simulink library "WECSim_Lib"  (R2014b)
settings: Solver=ode45  StartTime=0.0  StopTime=10.0  RelTol=1e-3
undefined symbols (not defined in the file): body, constraint, pto, simu, waves, X, Y, Z
libraries: nesl_utility x178, sm_lib x59, vrlib x12
(part 1 of 6)
settings Model: Creator=cmichel  LastModifiedBy=yyu

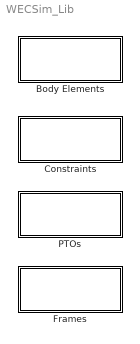
== system WECSim_Lib ==
  Body Elements : Subsystem
      mask Display: text(0,0,' ')
  Constraints : Subsystem
      mask Display: text(0,0,' ')
  Frames : Subsystem
      mask Display: text(0,0,' ')
  PTOs : Subsystem
      mask Display: text(0,0,' ')

== system WECSim_Lib/Body Elements ==
  Rigid Body : Subsystem  mask(BodyElements){body=body(1)}
      mask prompts: body "Body Name:"
      mask help: This block represents a rigid body. The variable name input below must be 'body(i)' where i=1,2,...
      mask init:
      | if exist('body','var')
      |     % geometry file name
      |     h=[gcb '/Structure/Body Properties'];
      |     geomFile=body.geometryFile;
      |     set_param(h,'ExtGeomFileName',geomFile);
      |     % toWorkSpace: outputs
      |     h=[gcb '/To Workspace'];
      |     responseName=['body' num2str(body.bodyNumber) '_out'];
      |     set_param(h,'VariableName',responseName);
      |     % toWorkSpace: hydrostatic pressures
      |     h=[gcb '/Hydrostatic Restoring Force Calculation/Linear and Nonlinear Restoring Force Variant Subsystem/Nonlinear Hydrostatic Restoring Force/To Workspace1'];
      |     responseName=['body' num2str(body.bodyNumber) '_hspressure_out'];
      |     set_param(h,'VariableName',responseName); 
      |     % toWorkSpace: wave pressures (non-linear Freude-Krylov)
      |     h=[gcb '/Wave Diffraction and Excitation Force Calculation/Nonlinear FK Force Variant Subsystem/With Nonlinear FroudeKrylov Force/To Workspace'];
      |     responseName=['body' num2str(body.bodyNumber) '_wavenonlinearpressure_out'];
      |     set_param(h,'VariableName',responseName);
      |     % toWorkSpace: wave pressures (linear Freude-Krylov)
      |     h=[gcb '/Wave Diffraction and Excitation Force Calculation/Nonlinear FK Force Variant Subsystem/With Nonlinear FroudeKrylov Force/To Workspace1'];
      |     responseName=['body' num2str(body.bodyNumber) '_wavelinearpressure_out'];
      |     set_param(h,'VariableName',responseName);
      |     % position GoTo 
      |     h=[gcb '/Goto'];
      |     responseName=['disp' num2str(body.bodyNumber)];
      |     set_param(h,'GotoTag',responseName);
      |     % position From
      |     h=[gcb '/From'];
      |     responseName=['disp' num2str(body.bodyNumber)];
      |     set_param(h,'GotoTag',responseName);
      |     % velocity GoTo 
      |     h=[gcb '/Goto1'];
      |     responseName=['vel' num2str(body.bodyNumber)];
      |     set_param(h,'GotoTag',responseName);
      |     % velocity From 
      |     h=[gcb '/From1'];
      |     responseName=['vel' num2str(body.bodyNumber)];
      |     set_param(h,'GotoTag',responseName);
      |     % acceleration GoTo 
      |     h=[gcb '/Goto2'];
      |     responseName=['acc' num2str(body.bodyNumber)];
      |     set_param(h,'GotoTag',responseName);
      |     % acceleration From 
      |     h=[gcb '/From2'];
      |     responseName=['acc' num2str(body.bodyNumber)];
      |     set_param(h,'GotoTag',responseName);
      | end
      | clear bc h geomFile responseName
      settings: AttributesFormatString=%<body>

== system WECSim_Lib/Constraints ==
  Fixed : Subsystem  mask(Constraints){constraint=constraint(1)}
      mask prompts: constraint "Constraint Name:"
      mask help:
      | Does not allow any motion. The variable name input below must be 'constraint(i)' where i=1,2,...
      |
      | constraint(i) must be defined in the input file with the following fields:
      |     .name              = a string
      |     .loc (optional)    = a 3x1 vector [x y z] in m. Default = [0 0 0]
      | The name string is used as the variable name for the output power and as such must comply with all of Matlab's variable naming rules.
      mask init:
      | if exist('constraint','var')
      |     h=[gcb '/output'];
      |     responseName=['constraint' num2str(constraint.constraintNum) '_out'];
      |     set_param(h,'VariableName',responseName);
      | end
      | 
      | constraint.checkLoc('W');
      settings: AttributesFormatString=%<constraint>
  Floating (3DOF) : Subsystem  mask(Constraints){constraint=constraint(1)}
      mask prompts: constraint "Constraint Name:"
      mask help:
      | Allows body to be free floating (motion in Surge, Heave, and Pitch). The variable name input below must be 'constraint(i)' where i=1,2,...
      |
      | constraint(i) must be defined in the input file with the following fields:
      |     .name              = a string
      |     .loc (optional)    = a 3x1 vector [x y z] in m. Default = [0 0 0]
      |
      | The name string is used as the variable name for the output power and as such must comply with all of Matlab's variable naming rules.
      mask init:
      | if exist('constraint','var')
      |     h=[gcb '/output'];
      |     responseName=['constraint' num2str(constraint.constraintNum) '_out'];
      |     set_param(h,'VariableName',responseName);
      | end
      | 
      | constraint.checkLoc('W');
      settings: AttributesFormatString=%<constraint>
  Floating (6DOF) : Subsystem  mask(Constraints){constraint=constraint(1)}
      mask prompts: constraint "Constraint Name:"
      mask help:
      | Allows body to be free floating (all 6 DOFs). The variable name input below must be 'constraint(i)' where i=1,2,...
      |
      | constraint(i) must be defined in the input file with the following fields:
      |     .name              = a string
      |     .loc (optional)    = a 3x1 vector [x y z] in m. Default = [0 0 0]
      |
      | The name string is used as the variable name for the output power and as such must comply with all of Matlab's variable naming rules.
      mask init: same as WECSim_Lib/Constraints/Floating (3DOF)
      settings: AttributesFormatString=%<constraint>
  Heave : Subsystem  mask(Constraints){constraint=constraint(1)}
      mask prompts: constraint "Constraint Name:"
      mask help:
      | Constrains motion to Heave translation only.The variable name input below must be 'constraint(i)' where i=1,2,...
      |
      | constraint(i) must be defined in the input file with the following fields:
      |     .name              = a string
      |     .loc (optional)    = a 3x1 vector [x y z] in m. Default = [0 0 0]
      | The name string is used as the variable name for the output power and as such must comply with all of Matlab's variable naming rules.
      mask init: same as WECSim_Lib/Constraints/Fixed
      settings: AttributesFormatString=%<constraint>
  Pitch : Subsystem  mask(Constraints){constraint=constraint(1)}
      mask prompts: constraint "Constraint Name:"
      mask help:
      | Constrains motion to Pitch rotation only. The variable name input below must be 'constraint(i)' where i=1,2,...
      |
      | constraint(i) must be defined in the input file with the following fields:
      |     .name   = a string
      |     .loc    = a 3x1 vector [x y z] in m
      |
      | The name string is used as the variable name for the output power and as such must comply with all of Matlab's variable naming rules.
      mask init:
      | if exist('constraint','var')
      |     h=[gcb '/output'];
      |     responseName=['constraint' num2str(constraint.constraintNum) '_out'];
      |     set_param(h,'VariableName',responseName);
      | end
      | 
      | constraint.checkLoc('E');
      settings: AttributesFormatString=%<constraint>
  Surge : Subsystem  mask(Constraints){constraint=constraint(1)}
      mask prompts: constraint "Constraint Name:"
      mask help:
      | Constrains motion to Surge translation only.The variable name input below must be 'constraint(i)' where i=1,2,...
      |
      | constraint(i) must be defined in the input file with the following fields:
      |     .name              = a string
      |     .loc (optional)    = a 3x1 vector [x y z] in m. Default = [0 0 0]
      |
      | The name string is used as the variable name for the output power and as such must comply with all of Matlab's variable naming rules.
      mask init: same as WECSim_Lib/Constraints/Fixed
      settings: AttributesFormatString=%<constraint>

== system WECSim_Lib/Frames ==
  Global Reference Frame : Subsystem  mask(Frames){waves=waves, simu=simu}
      mask prompts: waves "Wave Class Name"; simu "Simulation Class Name"
      mask help:
      | This block contains Global References, including solver configurations, free surface and seabed description, and simulation time.
      | It uses the following fields from the Simulation and Wave classes:
      |
      | Simulation Class:
      |     .endTime
      |     .dt
      |     .domainSize
      |
      | Wave Class:
      |     .waterDepth

== system WECSim_Lib/PTOs ==
  Rotational PTO (Local RY) : Subsystem  mask(PTO){pto=pto(1)}
      mask prompts: pto "PTO Name:"
      mask help:
      | This PTO constrains the follower (F) to only rotate about the Y-axis of the base (B), and applies a PTO stiffness and damping value. The variable name input below must be 'pto(i)' where i=1,2,...
      |
      | pto(i) must be defined in the input file with the following fields:
      |     .name   = a string
      |     .k      = a scalar in N*m/radians
      |     .c      = a scalar in N*m/(radians/s)
      |     .loc    = a 3x1 vector [x y z] in m
      |
      | The name string is used as the variable name for the output power and as such must comply with all of Matlab's variable naming rules.
      mask init:
      | if exist('pto','var')
      |     h=[gcb '/output'];
      |     responseName=['pto' num2str(pto.ptoNum) '_out'];
      |     set_param(h,'VariableName',responseName);
      | end
      | 
      | pto.checkLoc('E');
      settings: AttributesFormatString=%<pto>
  Rotational PTO Prescribed Motion (Local RY) : Subsystem  mask(PTO){pto=pto(1)}
      mask prompts: pto "PTO Name:"
      mask help:
      | This PTO constrains the follower (F) to only rotate about the Y-axis of the base (B), and applies a PTO stiffness and damping value. The variable name input below must be 'pto(i)' where i=1,2,...
      |
      | pto(i) must be defined in the input file with the following fields:
      |     .name   = a string
      |     .k      = a scalar in N*m/radians
      |     .c      = a scalar in N*m/(radians/s)
      |     .loc    = a 3x1 vector [x y z] in m
      |
      | The name string is used as the variable name for the output power and as such must comply with all of Matlab's variable naming rules.
      mask init:
      | if exist('pto','var')
      |     h=[gcb '/output'];
      |     responseName=['pto' num2str(pto.ptoNum) '_out'];
      |     set_param(h,'VariableName',responseName);
      | end
      | 
      | pto.checkLoc('E');
      settings: AttributesFormatString=%<pto>
  Rotational PTO UD Torque (Local RY) : Subsystem  mask(PTO){pto=pto(1)}
      mask prompts: pto "PTO Name:"
      mask help:
      | This PTO constrains the follower (F) to only rotate about the Y-axis of the base (B), and applies a PTO stiffness and damping value. The variable name input below must be 'pto(i)' where i=1,2,...
      |
      | pto(i) must be defined in the input file with the following fields:
      |     .name   = a string
      |     .k      = a scalar in N*m/radians
      |     .c      = a scalar in N*m/(radians/s)
      |     .loc    = a 3x1 vector [x y z] in m
      |
      | The name string is used as the variable name for the output power and as such must comply with all of Matlab's variable naming rules.
      mask init:
      | if exist('pto','var')
      |     h=[gcb '/output'];
      |     responseName=['pto' num2str(pto.ptoNum) '_out'];
      |     set_param(h,'VariableName',responseName);
      | end
      | 
      | pto.checkLoc('E');
      settings: AttributesFormatString=%<pto>
  Translational PTO (Local X) : Subsystem  mask(PTO){pto=pto(1)}
      mask prompts: pto "PTO Name:"
      mask help:
      | This PTO constrains the follower (F) to only move along the X-direction of the base (B), and applies a PTO stiffness and damping value. The variable name input below must be 'pto(i)' where i=1,2,...
      |
      | pto(i) must be defined in the input file with the following fields:
      |     .name              = a string
      |     .k                 = a scalar in N/m
      |     .c                 = a scalar in N/(m/s)
      |     .loc (optional)    = a 3x1 vector [x y z] in m. Default = [0 0 0]
      | The name string is used as the variable name for the output power and as such must comply with all of Matlab's variable naming rules.
      mask init:
      | if exist('pto','var')
      |     h=[gcb '/output'];
      |     responseName=['pto' num2str(pto.ptoNum) '_out'];
      |     set_param(h,'VariableName',responseName);
      | end
      | 
      | pto.checkLoc('W');
      settings: AttributesFormatString=%<pto>
  Translational PTO (Local Z) : Subsystem  mask(PTO){pto=pto(1)}
      mask prompts: pto "PTO Name:"
      mask help:
      | This PTO constrains the follower (F) to only move along the Z-direction of the base (B), and applies a PTO stiffness and damping value. The variable name input below must be 'pto(i)' where i=1,2,...
      |
      | pto(i) must be defined in the input file with the following fields:
      |     .name               = a string
      |     .k                  = a scalar in N/m
      |     .c                  = a scalar in N/(m/s)
      |     .loc (optional)     = a 3x1 vector [x y z] in m. Default = [0 0 0]
      |
      | The name string is used as the variable name for the output power and as such must comply with all of Matlab's variable naming rules.
      mask init:
      | if exist('pto','var')
      |     h=[gcb '/output'];
      |     responseName=['pto' num2str(pto.ptoNum) '_out'];
      |     set_param(h,'VariableName',responseName);
      | end
      | 
      | pto.checkLoc('W');
      settings: AttributesFormatString=%<pto>
  Translational PTO Prescribed Motion (Local X) : Subsystem  mask(PTO){pto=pto(1)}
      mask prompts: pto "PTO Name:"
      mask help:
      | This PTO constrains the follower (F) to only move along the X-direction of the base (B), and applies a PTO stiffness and damping value. The variable name input below must be 'pto(i)' where i=1,2,...
      |
      | pto(i) must be defined in the input file with the following fields:
      |     .name              = a string
      |     .k                 = a scalar in N/m
      |     .c                 = a scalar in N/(m/s)
      |     .loc (optional)    = a 3x1 vector [x y z] in m. Default = [0 0 0]
      | The name string is used as the variable name for the output power and as such must comply with all of Matlab's variable naming rules.
      mask init:
      | if exist('pto','var')
      |     h=[gcb '/output'];
      |     responseName=['pto' num2str(pto.ptoNum) '_out'];
      |     set_param(h,'VariableName',responseName);
      | end
      | 
      | pto.checkLoc('W');
      settings: AttributesFormatString=%<pto>
  Translational PTO Prescribed Motion (Local Z) : Subsystem  mask(PTO){pto=pto(1)}
      mask prompts: pto "PTO Name:"
      mask help:
      | This PTO constrains the follower (F) to only move along the Z-direction of the base (B), and applies a PTO stiffness and damping value. The variable name input below must be 'pto(i)' where i=1,2,...
      |
      | pto(i) must be defined in the input file with the following fields:
      |     .name               = a string
      |     .k                  = a scalar in N/m
      |     .c                  = a scalar in N/(m/s)
      |     .loc (optional)     = a 3x1 vector [x y z] in m. Default = [0 0 0]
      |
      | The name string is used as the variable name for the output power and as such must comply with all of Matlab's variable naming rules.
      mask init:
      | if exist('pto','var')
      |     h=[gcb '/output'];
      |     responseName=['pto' num2str(pto.ptoNum) '_out'];
      |     set_param(h,'VariableName',responseName);
      | end
      | 
      | pto.checkLoc('W');
      settings: AttributesFormatString=%<pto>
  Translational PTO UD Force (Local X) : Subsystem  mask(PTO){pto=pto(1)}
      mask prompts: pto "PTO Name:"
      mask help:
      | This PTO constrains the follower (F) to only move along the X-direction of the base (B), and applies a PTO stiffness and damping value. The variable name input below must be 'pto(i)' where i=1,2,...
      |
      | pto(i) must be defined in the input file with the following fields:
      |     .name              = a string
      |     .k                 = a scalar in N/m
      |     .c                 = a scalar in N/(m/s)
      |     .loc (optional)    = a 3x1 vector [x y z] in m. Default = [0 0 0]
      | The name string is used as the variable name for the output power and as such must comply with all of Matlab's variable naming rules.
      mask init:
      | if exist('pto','var')
      |     h=[gcb '/output'];
      |     responseName=['pto' num2str(pto.ptoNum) '_out'];
      |     set_param(h,'VariableName',responseName);
      | end
      | 
      | pto.checkLoc('W');
      settings: AttributesFormatString=%<pto>
  Translational PTO UD Force (Local Z) : Subsystem  mask(PTO){pto=pto(1)}
      mask prompts: pto "PTO Name:"
      mask help:
      | This PTO constrains the follower (F) to only move along the Z-direction of the base (B), and applies a PTO stiffness and damping value. The variable name input below must be 'pto(i)' where i=1,2,...
      |
      | pto(i) must be defined in the input file with the following fields:
      |     .name               = a string
      |     .k                  = a scalar in N/m
      |     .c                  = a scalar in N/(m/s)
      |     .loc (optional)     = a 3x1 vector [x y z] in m. Default = [0 0 0]
      |
      | The name string is used as the variable name for the output power and as such must comply with all of Matlab's variable naming rules.
      mask init:
      | if exist('pto','var')
      |     h=[gcb '/output'];
      |     responseName=['pto' num2str(pto.ptoNum) '_out'];
      |     set_param(h,'VariableName',responseName);
      | end
      | 
      | pto.checkLoc('W');
      settings: AttributesFormatString=%<pto>

== system WECSim_Lib/Body Elements/Rigid Body ==
  note: body.hydroData.properties.name used in mask
  note: Calculates forces at the cg and applies it to the structure at the cg. Output results.
  Additional Linear Damping Force Calculation : Subsystem
  B2B Subsystem : Subsystem  Variant=on
  Bus Creator : BusCreator  Inputs=7
  Bus Creator1 : BusCreator  Inputs=3
  Bus Selector1 : BusSelector  OutputSignals=F_Excitation,F_RadiationDamping,F_AddedMass,F_Restoring,F_MorrisonAndViscous,F_Mooring,F_LinearDamping
  Bus Selector2 : BusSelector  OutputSignals=disp,vel,acc
  Hydrostatic Restoring Force Calculation : Subsystem
  Mooring Force Calculation (Map) : Subsystem
  Morrison Element and ViscousDampingForceCalculation : Subsystem
  Nonlinear Wave Elevation : Subsystem
  Structure : Subsystem
  Sum : Sum  Inputs=+------
  To Workspace : ToWorkspace  VariableName=body1_out  SaveFormat=Structure With Time  SampleTime=-1
      settings: Decimation=round(simu.dtOut/simu.dt,0)
  Wave Diffraction and Excitation Force Calculation : Subsystem
  Wave Radiation Forces Calculation : Subsystem
  Conn : PMIOPort  Port=1  Side=Right
  tag scope: acc1=global, disp1=global, vel1=global
  wires:
  [Clock] -> Wave Radiation Forces Calculation/3(Time), Hydrostatic Restoring Force Calculation/3(Time), Wave Diffraction and Excitation Force Calculation/1(Time), Nonlinear Wave Elevation/2(Time)
  Bus Selector1/7 -> Sum/7  "<F_LinearDamping>"
  Bus Selector1/1 -> Sum/1  "<F_Excitation>"
  Bus Selector1/6 -> Sum/6  "<F_Mooring>"
  Bus Selector1/2 -> Sum/2  "<F_RadiationDamping>"
  Bus Selector1/5 -> Sum/5  "<F_MorrisonAndViscous>"
  Bus Selector1/3 -> Sum/3  "<F_AddedMass>"
  Bus Selector1/4 -> Sum/4  "<F_Restoring>"
  Wave Radiation Forces Calculation/2(F_AddedMass) -> Bus Creator/3
  Additional Linear Damping Force Calculation/1(F_LinearDamping) -> Bus Creator/7
  Wave Diffraction and Excitation Force Calculation/1(F_Excitation) -> Bus Creator/1
  Wave Radiation Forces Calculation/1(F_RadiationDamping) -> Bus Creator/2
  Hydrostatic Restoring Force Calculation/1(F_Restoring) -> Bus Creator/4
  Morrison Element and ViscousDampingForceCalculation/1(F_MorrisonAndViscous) -> Bus Creator/5
  Mooring Force Calculation (Map)/1(F_Mooring) -> Bus Creator/6
  Bus Creator1/1 -> To Workspace/1
  Bus Creator/1 -> Bus Selector1/1, Bus Creator1/3  "BUS(7): Forces"
  Sum/1 -> Structure/1(Total Force), Bus Creator1/2  "F_Total"
  Nonlinear Wave Elevation/1(Wave Elevation) -> Hydrostatic Restoring Force Calculation/2(Wave Elv), Wave Diffraction and Excitation Force Calculation/3(WaveElv)
  [vel1] -> B2B Subsystem/1(vel_in), Morrison Element and ViscousDampingForceCalculation/3(Velocity), Mooring Force Calculation (Map)/2(Velocity), Additional Linear Damping Force Calculation/1(Velocity)
  [acc1] -> Morrison Element and ViscousDampingForceCalculation/2(Acceleration), B2B Subsystem/2(acc_in)
  [disp1] -> Wave Diffraction and Excitation Force Calculation/2(Displacement), Nonlinear Wave Elevation/1(Displacement), Morrison Element and ViscousDampingForceCalculation/1(Displacement), Mooring Force Calculation (Map)/1(Displacement), Hydrostatic Restoring Force Calculation/1(Displacement)
  B2B Subsystem/1(vel) -> Wave Radiation Forces Calculation/1(Velocity)
  B2B Subsystem/2(acc) -> Wave Radiation Forces Calculation/2(Acceleration)
  Structure/1(Response) -> Bus Selector2/1, Bus Creator1/1
  Bus Selector2/2 -> [vel1]  "<vel>"
  Bus Selector2/3 -> [acc1]  "<acc>"
  Bus Selector2/1 -> [disp1]  "<disp>"
  connections:
  Conn/RConn1 -- Structure/RConn1

== system WECSim_Lib/Constraints/Fixed ==
  note: Constraints the motion to the desired DOF.
      | Moves the connection points (B and F) from the free surface to the PTO location.
      | Outputs forces and motions.
  note: constraint.loc
      | constraint.c
      | constraint.k
      | constraint.name used in mask
  Constant{,1..3} (4 alike) : Constant  Value=[0 0 0 0 0 0]
  Mux : Mux  Inputs=2
  Mux1 : Mux  Inputs=6
  Mux2 : Mux  Inputs=2
  PS-Simulink Converter{,1..3} (4 alike) : nesl_utility/PS-Simulink Converter  PhysicalDomain=network_engine_domain  SubClassName=ps_output  LeftPortType=input  RightPortType=output  PseudoPeriodic=off  Frequencies=[]  Unit=1  AffineConversion=off
  Rigid Transform : sm_lib/Frames and Transforms/Rigid Transform  TranslationMethod=Cartesian  TranslationLengthUnit=m  TranslationStandardAxis=+Z  TranslationStandardOffset=0  TranslationCartesianOffset=constraint.loc  TranslationROffset=0  TranslationROffsetUnits=m  TranslationZOffset=0  TranslationZOffsetUnits=m  TranslationThetaOffset=0  TranslationThetaOffsetUnits=deg  RotationMethod=None  RotationAngleUnits=deg  RotationStandardAxis=+X  RotationAngle=90  RotationArbitraryAxis=[0 0 1]  FollAlignAxisA=+X  BaseAlignAxisA=+Y  FollAlignAxisB=+Y  BaseAlignAxisB=+Z  RotationMatrix=[1 0 0; 0 1 0; 0 0 1]  BlockFunction=simmechanics.library.frames_transforms.rigid_transform
  Rigid Transform1 : sm_lib/Frames and Transforms/Rigid Transform  TranslationMethod=Cartesian  TranslationLengthUnit=m  TranslationStandardAxis=+Z  TranslationStandardOffset=0  TranslationCartesianOffset=constraint.loc  TranslationROffset=0  TranslationROffsetUnits=m  TranslationZOffset=0  TranslationZOffsetUnits=m  TranslationThetaOffset=0  TranslationThetaOffsetUnits=deg  RotationMethod=None  RotationAngleUnits=deg  RotationStandardAxis=+X  RotationAngle=90  RotationArbitraryAxis=[0 0 1]  FollAlignAxisA=+X  BaseAlignAxisA=+Y  FollAlignAxisB=+Y  BaseAlignAxisB=+Z  RotationMatrix=[1 0 0; 0 1 0; 0 0 1]  BlockFunction=simmechanics.library.frames_transforms.rigid_transform
  Weld Joint (Fixed) : sm_lib/Joints/Weld Joint  SenseConstraintForce=on  SenseConstraintForceX=off  SenseConstraintForceY=off  SenseConstraintForceZ=off  SenseConstraintTorque=on  SenseConstraintTorqueX=off  SenseConstraintTorqueY=off  SenseConstraintTorqueZ=off  SenseTotalForce=on  SenseTotalForceX=off  SenseTotalForceY=off  SenseTotalForceZ=off  SenseTotalTorque=on  SenseTotalTorqueX=off  SenseTotalTorqueY=off  SenseTotalTorqueZ=off  CompositeWrenchDir=BaseOnFollower  CompositeWrenchFrame=BaseFrame  BlockFunction=simmechanics.library.joints.weld_joint
  output : ToWorkspace  VariableName=constraint1_out  SaveFormat=Structure With Time  SampleTime=-1
      settings: Decimation=round(simu.dtOut/simu.dt,0)
  B : PMIOPort  Port=1  Side=Left
  F : PMIOPort  Port=2  Side=Right
  wires:
  Constant2/1 -> Mux1/3  "acceleration"
  Constant1/1 -> Mux1/2  "velocity"
  Constant/1 -> Mux1/1  "position"
  Mux1/1 -> output/1
  Mux/1 -> Mux1/5  "Constraint Forces"
  PS-Simulink Converter1/1 -> Mux/2
  PS-Simulink Converter/1 -> Mux/1
  Constant3/1 -> Mux1/6  "Mooring Forces"
  Mux2/1 -> Mux1/4  "Total Forces"
  PS-Simulink Converter3/1 -> Mux2/2
  PS-Simulink Converter2/1 -> Mux2/1
  connections:
  Rigid Transform/LConn1 -- B/RConn1
  Weld Joint (Fixed)/LConn1 -- Rigid Transform/RConn1
  Rigid Transform1/RConn1 -- Weld Joint (Fixed)/RConn1
  F/RConn1 -- Rigid Transform1/LConn1
  PS-Simulink Converter/LConn1 -- Weld Joint (Fixed)/RConn2
  PS-Simulink Converter1/LConn1 -- Weld Joint (Fixed)/RConn3
  PS-Simulink Converter2/LConn1 -- Weld Joint (Fixed)/RConn4
  PS-Simulink Converter3/LConn1 -- Weld Joint (Fixed)/RConn5

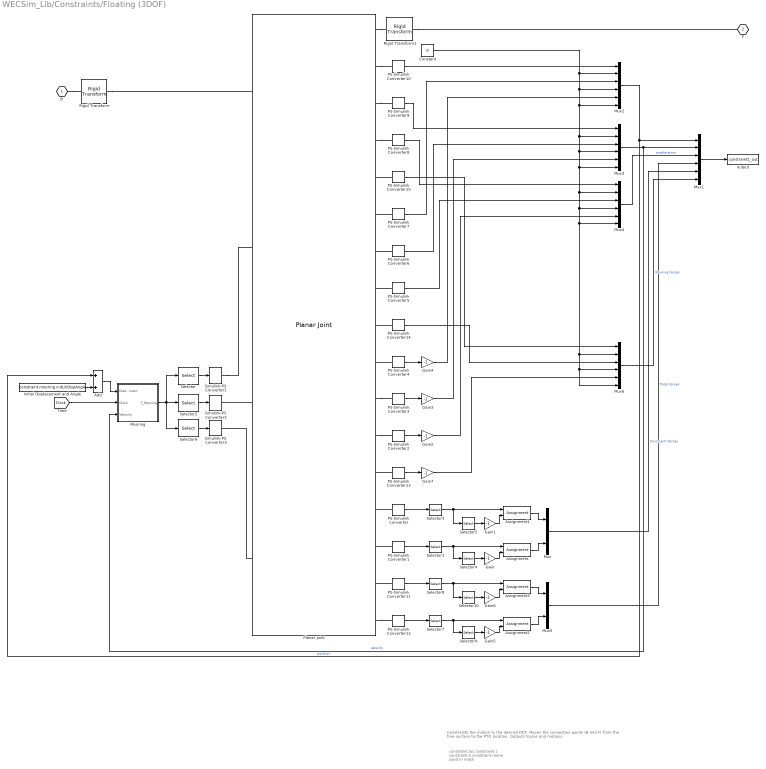
== system WECSim_Lib/Constraints/Floating (3DOF) ==
  note: Constraints the motion to the desired DOF.
      | Moves the connection points (B and F) from the free surface to the PTO location.
      | Outputs forces and motions.
  note: constraint.loc
      | constraint.c
      | constraint.k
      | constraint.name used in mask
  Add : Sum
  Assignment{,1..3} (4 alike) : Assignment  DiagnosticForDimensions=Warning  Indices=2
  Constant : Constant  Value=0
  Gain{,1..7} (8 alike) : Gain  Gain=-1
  Initial Displacement and Angle : Constant  Value=constraint.mooring.initLinDispAngle
  Mooring : Subsystem  Variant=on
  Mux : Mux  Inputs=2
  Mux{1..4,6} (5 alike) : Mux  Inputs=6
  Mux5 : Mux  Inputs=2
  PS-Simulink Converter{,1..15} (16 alike) : nesl_utility/PS-Simulink Converter  PhysicalDomain=network_engine_domain  SubClassName=ps_output  LeftPortType=input  RightPortType=output  PseudoPeriodic=off  Frequencies=[]  Unit=1  AffineConversion=off
  Planar Joint : sm_lib/Joints/Planar Joint  SenseConstraintForce=on  SenseConstraintForceX=off  SenseConstraintForceY=off  SenseConstraintForceZ=off  SenseConstraintTorque=on  SenseConstraintTorqueX=off  SenseConstraintTorqueY=off  SenseConstraintTorqueZ=off  SenseTotalForce=on  SenseTotalForceX=off  SenseTotalForceY=off  SenseTotalForceZ=off  SenseTotalTorque=on  SenseTotalTorqueX=off  SenseTotalTorqueY=off  SenseTotalTorqueZ=off  CompositeWrenchDir=BaseOnFollower  CompositeWrenchFrame=BaseFrame  PxEquilibriumPosition=0  PxEquilibriumPositionUnits=m  PxSpringStiffness=0  PxSpringStiffnessUnits=N/m  PxDampingCoefficient=0  PxDampingCoefficientUnits=N/(m/s)  PxTorqueActuationMode=InputTorque  PxMotionActuationMode=ComputedMotion  PxSensePosition=on  PxSenseVelocity=on  PxSenseAcceleration=on  PxSenseTorqueForce=on  PxPositionTargetValue=0  PxPositionTargetValueUnits=m  PxPositionTargetSpecify=off  PxPositionTargetPriority=High  PxVelocityTargetValue=0  PxVelocityTargetValueUnits=m/s  PxVelocityTargetSpecify=off  PxVelocityTargetPriority=High  PyEquilibriumPosition=0  PyEquilibriumPositionUnits=m  PySpringStiffness=0  PySpringStiffnessUnits=N/m  PyDampingCoefficient=0  PyDampingCoefficientUnits=N/(m/s)  PyTorqueActuationMode=InputTorque  PyMotionActuationMode=ComputedMotion  PySensePosition=on  PySenseVelocity=on  PySenseAcceleration=on  PySenseTorqueForce=on  PyPositionTargetValue=0  PyPositionTargetValueUnits=m  PyPositionTargetSpecify=off  PyPositionTargetPriority=High  PyVelocityTargetValue=0  PyVelocityTargetValueUnits=m/s  PyVelocityTargetSpecify=off  PyVelocityTargetPriority=High  RzEquilibriumPosition=0  RzEquilibriumPositionUnits=deg  RzSpringStiffness=0  RzSpringStiffnessUnits=N*m/deg  RzDampingCoefficient=0  RzDampingCoefficientUnits=N*m/(deg/s)  RzTorqueActuationMode=InputTorque  RzMotionActuationMode=ComputedMotion  RzSensePosition=on  RzSenseVelocity=on  RzSenseAcceleration=on  RzSenseTorqueForce=on  RzPositionTargetValue=0  RzPositionTargetValueUnits=deg  RzPositionTargetSpecify=off  RzPositionTargetPriority=High  RzVelocityTargetValue=0  RzVelocityTargetValueUnits=deg/s  RzVelocityTargetSpecify=off  RzVelocityTargetPriority=High  BlockFunction=simmechanics.library.joints.planar_joint
  Rigid Transform : sm_lib/Frames and Transforms/Rigid Transform  TranslationMethod=Cartesian  TranslationLengthUnit=m  TranslationStandardAxis=+Z  TranslationStandardOffset=0  TranslationCartesianOffset=constraint.loc  TranslationROffset=0  TranslationROffsetUnits=m  TranslationZOffset=0  TranslationZOffsetUnits=m  TranslationThetaOffset=0  TranslationThetaOffsetUnits=deg  RotationMethod=StandardAxis  RotationAngleUnits=deg  RotationStandardAxis=+X  RotationAngle=90  RotationArbitraryAxis=[0 0 1]  FollAlignAxisA=+X  BaseAlignAxisA=+Y  FollAlignAxisB=+Y  BaseAlignAxisB=+Z  RotationMatrix=[1 0 0; 0 1 0; 0 0 1]  BlockFunction=simmechanics.library.frames_transforms.rigid_transform
  Rigid Transform1 : sm_lib/Frames and Transforms/Rigid Transform  TranslationMethod=Cartesian  TranslationLengthUnit=m  TranslationStandardAxis=+Z  TranslationStandardOffset=0  TranslationCartesianOffset=constraint.loc  TranslationROffset=0  TranslationROffsetUnits=m  TranslationZOffset=0  TranslationZOffsetUnits=m  TranslationThetaOffset=0  TranslationThetaOffsetUnits=deg  RotationMethod=StandardAxis  RotationAngleUnits=deg  RotationStandardAxis=+X  RotationAngle=90  RotationArbitraryAxis=[0 0 1]  FollAlignAxisA=+X  BaseAlignAxisA=+Y  FollAlignAxisB=+Y  BaseAlignAxisB=+Z  RotationMatrix=[1 0 0; 0 1 0; 0 0 1]  BlockFunction=simmechanics.library.frames_transforms.rigid_transform
  Selector : Selector  InputPortWidth=6
  Selector{1,3,7..8} (4 alike) : Selector  InputPortWidth=3  Indices=[1 3 2]
  Selector{4..5,9..10} (4 alike) : Selector  InputPortWidth=3  Indices=[2]
  Selector2 : Selector  InputPortWidth=6  Indices=3
  Selector6 : Selector  InputPortWidth=6  Indices=5
  Simulink-PS Converter1 : nesl_utility/Simulink-PS Converter  PhysicalDomain=network_engine_domain  SubClassName=ps_input  LeftPortType=input  RightPortType=output  PseudoPeriodic=off  Frequencies=[]  NoiseDistribution=none  NoiseParameters=[]  Unit=1  AffineConversion=off  InputFiltering=off  SimscapeFilterOrder=1  InputFilterTimeConstant=0.001  UdotUserProvided=1
  Simulink-PS Converter2 : nesl_utility/Simulink-PS Converter  PhysicalDomain=network_engine_domain  SubClassName=ps_input  LeftPortType=input  RightPortType=output  PseudoPeriodic=off  Frequencies=[]  NoiseDistribution=none  NoiseParameters=[]  Unit=1  AffineConversion=off  InputFiltering=off  SimscapeFilterOrder=1  InputFilterTimeConstant=0.001  UdotUserProvided=1
  Simulink-PS Converter3 : nesl_utility/Simulink-PS Converter  PhysicalDomain=network_engine_domain  SubClassName=ps_input  LeftPortType=input  RightPortType=output  PseudoPeriodic=off  Frequencies=[]  NoiseDistribution=none  NoiseParameters=[]  Unit=1  AffineConversion=off  InputFiltering=off  SimscapeFilterOrder=1  InputFilterTimeConstant=0.001  UdotUserProvided=1
  output : ToWorkspace  VariableName=constraint1_out  SaveFormat=Structure With Time  SampleTime=-1
      settings: Decimation=round(simu.dtOut/simu.dt,0)
  B : PMIOPort  Port=1  Side=Left
  F : PMIOPort  Port=2  Side=Right
  wires:
  Gain2/1 -> Mux4/5
  Gain3/1 -> Mux3/5
  Gain4/1 -> Mux2/5
  PS-Simulink Converter2/1 -> Gain2/1
  PS-Simulink Converter3/1 -> Gain3/1
  PS-Simulink Converter4/1 -> Gain4/1
  PS-Simulink Converter5/1 -> Mux4/3
  PS-Simulink Converter6/1 -> Mux3/3
  PS-Simulink Converter7/1 -> Mux2/3
  Constant/1 -> Mux6/2, Mux6/4, Mux6/6, Mux4/6, Mux4/4, Mux4/2, Mux3/6, Mux3/4, Mux3/2, Mux2/6, Mux2/4, Mux2/2
  PS-Simulink Converter8/1 -> Mux4/1
  PS-Simulink Converter9/1 -> Mux3/1
  PS-Simulink Converter10/1 -> Mux2/1
  Mux4/1 -> Mux1/3  "acceleration"
  Mux3/1 -> Mux1/2, Mooring/3(Velocity)  "velocity"
  Mux2/1 -> Add/1, Mux1/1  "position"
  Mux1/1 -> output/1
  Assignment1/1 -> Mux/1
  Assignment/1 -> Mux/2
  PS-Simulink Converter/1 -> Selector3/1
  PS-Simulink Converter1/1 -> Selector1/1
  Gain1/1 -> Assignment1/2
  Selector5/1 -> Gain1/1
  Selector3/1 -> Selector5/1, Assignment1/1
  Gain/1 -> Assignment/2
  Selector4/1 -> Gain/1
  Selector1/1 -> Selector4/1, Assignment/1
  Mux/1 -> Mux1/5  "Constraint Forces"
  Mooring/1(F_Mooring) -> Selector/1, Selector2/1, Selector6/1
  Selector/1 -> Simulink-PS Converter1/1
  Selector2/1 -> Simulink-PS Converter2/1
  Selector6/1 -> Simulink-PS Converter3/1
  [Clock] -> Mooring/2(Clock)
  Assignment3/1 -> Mux5/1
  Assignment2/1 -> Mux5/2
  PS-Simulink Converter11/1 -> Selector8/1
  PS-Simulink Converter12/1 -> Selector7/1
  Gain6/1 -> Assignment3/2
  Selector10/1 -> Gain6/1
  Selector8/1 -> Selector10/1, Assignment3/1
  Gain5/1 -> Assignment2/2
  Selector9/1 -> Gain5/1
  Selector7/1 -> Selector9/1, Assignment2/1
  Mux5/1 -> Mux1/4  "Total Forces"
  PS-Simulink Converter13/1 -> Gain7/1
  Gain7/1 -> Mux6/5
  PS-Simulink Converter14/1 -> Mux6/3
  PS-Simulink Converter15/1 -> Mux6/1
  Mux6/1 -> Mux1/6  "Mooring Forces"
  Initial Displacement and Angle/1 -> Add/2
  Add/1 -> Mooring/1(Displacement)
  connections:
  Planar Joint/RConn4 -- PS-Simulink Converter8/LConn1
  Planar Joint/RConn3 -- PS-Simulink Converter9/LConn1
  Planar Joint/RConn2 -- PS-Simulink Converter10/LConn1
  B/RConn1 -- Rigid Transform/LConn1
  Rigid Transform/RConn1 -- Planar Joint/LConn1
  Planar Joint/RConn1 -- Rigid Transform1/RConn1
  Rigid Transform1/LConn1 -- F/RConn1
  Simulink-PS Converter1/RConn1 -- Planar Joint/LConn2
  Planar Joint/LConn3 -- Simulink-PS Converter2/RConn1
  Planar Joint/LConn4 -- Simulink-PS Converter3/RConn1
  PS-Simulink Converter/LConn1 -- Planar Joint/RConn14
  PS-Simulink Converter1/LConn1 -- Planar Joint/RConn15
  Planar Joint/RConn17 -- PS-Simulink Converter12/LConn1
  PS-Simulink Converter11/LConn1 -- Planar Joint/RConn16
  PS-Simulink Converter7/LConn1 -- Planar Joint/RConn6
  PS-Simulink Converter6/LConn1 -- Planar Joint/RConn7
  PS-Simulink Converter5/LConn1 -- Planar Joint/RConn8
  PS-Simulink Converter4/LConn1 -- Planar Joint/RConn10
  Planar Joint/RConn11 -- PS-Simulink Converter3/LConn1
  Planar Joint/RConn12 -- PS-Simulink Converter2/LConn1
  PS-Simulink Converter13/LConn1 -- Planar Joint/RConn13
  PS-Simulink Converter14/LConn1 -- Planar Joint/RConn9
  PS-Simulink Converter15/LConn1 -- Planar Joint/RConn5

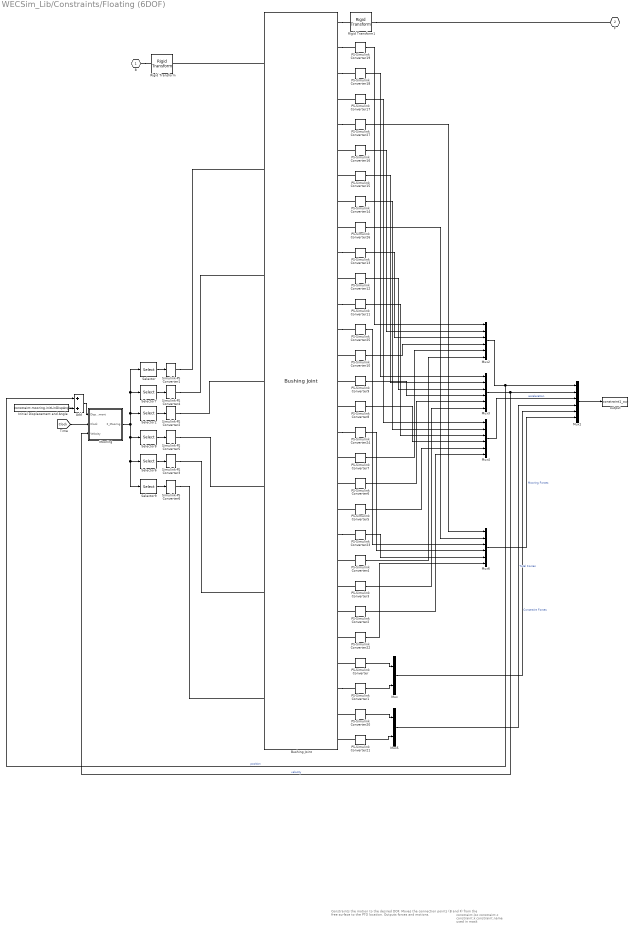
== system WECSim_Lib/Constraints/Floating (6DOF) ==
  note: constraint.loc
      | constraint.c
      | constraint.k
      | constraint.name used in mask
  note: Constraints the motion to the desired DOF.
      | Moves the connection points (B and F) from the free surface to the PTO location.
      | Outputs forces and motions.
  Add : Sum
  Bushing Joint : sm_lib/Joints/Bushing Joint  SenseConstraintForce=on  SenseConstraintForceX=off  SenseConstraintForceY=off  SenseConstraintForceZ=off  SenseConstraintTorque=on  SenseConstraintTorqueX=off  SenseConstraintTorqueY=off  SenseConstraintTorqueZ=off  SenseTotalForce=on  SenseTotalForceX=off  SenseTotalForceY=off  SenseTotalForceZ=off  SenseTotalTorque=on  SenseTotalTorqueX=off  SenseTotalTorqueY=off  SenseTotalTorqueZ=off  CompositeWrenchDir=BaseOnFollower  CompositeWrenchFrame=BaseFrame  PxEquilibriumPosition=0  PxEquilibriumPositionUnits=m  PxSpringStiffness=0  PxSpringStiffnessUnits=N/m  PxDampingCoefficient=0  PxDampingCoefficientUnits=N/(m/s)  PxTorqueActuationMode=InputTorque  PxMotionActuationMode=ComputedMotion  PxSensePosition=on  PxSenseVelocity=on  PxSenseAcceleration=on  PxSenseTorqueForce=on  PxPositionTargetValue=0  PxPositionTargetValueUnits=m  PxPositionTargetSpecify=off  PxPositionTargetPriority=High  PxVelocityTargetValue=0  PxVelocityTargetValueUnits=m/s  PxVelocityTargetSpecify=off  PxVelocityTargetPriority=High  PyEquilibriumPosition=0  PyEquilibriumPositionUnits=m  PySpringStiffness=0  PySpringStiffnessUnits=N/m  PyDampingCoefficient=0  PyDampingCoefficientUnits=N/(m/s)  PyTorqueActuationMode=InputTorque  PyMotionActuationMode=ComputedMotion  PySensePosition=on  PySenseVelocity=on  PySenseAcceleration=on  PySenseTorqueForce=on  PyPositionTargetValue=0  PyPositionTargetValueUnits=m  PyPositionTargetSpecify=off  PyPositionTargetPriority=High  PyVelocityTargetValue=0  PyVelocityTargetValueUnits=m/s  PyVelocityTargetSpecify=off  PyVelocityTargetPriority=High  PzEquilibriumPosition=0  PzEquilibriumPositionUnits=m  PzSpringStiffness=0  PzSpringStiffnessUnits=N/m  PzDampingCoefficient=0  PzDampingCoefficientUnits=N/(m/s)  PzTorqueActuationMode=InputTorque  PzMotionActuationMode=ComputedMotion  PzSensePosition=on  PzSenseVelocity=on  PzSenseAcceleration=on  PzSenseTorqueForce=on  PzPositionTargetValue=0  PzPositionTargetValueUnits=m  PzPositionTargetSpecify=off  PzPositionTargetPriority=High  PzVelocityTargetValue=0  PzVelocityTargetValueUnits=m/s  PzVelocityTargetSpecify=off  PzVelocityTargetPriority=High  RxEquilibriumPosition=0  RxEquilibriumPositionUnits=deg  RxSpringStiffness=0  RxSpringStiffnessUnits=N*m/deg  RxDampingCoefficient=0  RxDampingCoefficientUnits=N*m/(deg/s)  RxTorqueActuationMode=InputTorque  RxMotionActuationMode=ComputedMotion  RxSensePosition=on  RxSenseVelocity=on  RxSenseAcceleration=on  RxSenseTorqueForce=on  RxPositionTargetValue=0  RxPositionTargetValueUnits=deg  RxPositionTargetSpecify=off  RxPositionTargetPriority=High  RxVelocityTargetValue=0  RxVelocityTargetValueUnits=deg/s  RxVelocityTargetSpecify=off  RxVelocityTargetPriority=High  RyEquilibriumPosition=0  RyEquilibriumPositionUnits=deg  RySpringStiffness=0  RySpringStiffnessUnits=N*m/deg  RyDampingCoefficient=0  RyDampingCoefficientUnits=N*m/(deg/s)  RyTorqueActuationMode=InputTorque  RyMotionActuationMode=ComputedMotion  RySensePosition=on  RySenseVelocity=on  RySenseAcceleration=on  RySenseTorqueForce=on  RyPositionTargetValue=0  RyPositionTargetValueUnits=deg  RyPositionTargetSpecify=off  RyPositionTargetPriority=High  RyVelocityTargetValue=0  RyVelocityTargetValueUnits=deg/s  RyVelocityTargetSpecify=off  RyVelocityTargetPriority=High  RzEquilibriumPosition=0  RzEquilibriumPositionUnits=deg  RzSpringStiffness=0  RzSpringStiffnessUnits=N*m/deg  RzDampingCoefficient=0  RzDampingCoefficientUnits=N*m/(deg/s)  RzTorqueActuationMode=InputTorque  RzMotionActuationMode=ComputedMotion  RzSensePosition=on  RzSenseVelocity=on  RzSenseAcceleration=on  RzSenseTorqueForce=on  RzPositionTargetValue=0  RzPositionTargetValueUnits=deg  RzPositionTargetSpecify=off  RzPositionTargetPriority=High  RzVelocityTargetValue=0  RzVelocityTargetValueUnits=deg/s  RzVelocityTargetSpecify=off  RzVelocityTargetPriority=High  BlockFunction=simmechanics.library.joints.bushing_joint
  Initial Displacement and Angle : Constant  Value=constraint.mooring.initLinDispAngle
  Mooring : Subsystem  Variant=on
  Mux : Mux  Inputs=2
  Mux{1..4,6} (5 alike) : Mux  Inputs=6
  Mux5 : Mux  Inputs=2
  PS-Simulink Converter{,1..27} (28 alike) : nesl_utility/PS-Simulink Converter  PhysicalDomain=network_engine_domain  SubClassName=ps_output  LeftPortType=input  RightPortType=output  PseudoPeriodic=off  Frequencies=[]  Unit=1  AffineConversion=off
  Rigid Transform : sm_lib/Frames and Transforms/Rigid Transform  TranslationMethod=Cartesian  TranslationLengthUnit=m  TranslationStandardAxis=+Z  TranslationStandardOffset=0  TranslationCartesianOffset=constraint.loc  TranslationROffset=0  TranslationROffsetUnits=m  TranslationZOffset=0  TranslationZOffsetUnits=m  TranslationThetaOffset=0  TranslationThetaOffsetUnits=deg  RotationMethod=None  RotationAngleUnits=deg  RotationStandardAxis=+X  RotationAngle=90  RotationArbitraryAxis=[0 0 1]  FollAlignAxisA=+X  BaseAlignAxisA=+Y  FollAlignAxisB=+Y  BaseAlignAxisB=+Z  RotationMatrix=[1 0 0; 0 1 0; 0 0 1]  BlockFunction=simmechanics.library.frames_transforms.rigid_transform
  Rigid Transform1 : sm_lib/Frames and Transforms/Rigid Transform  TranslationMethod=Cartesian  TranslationLengthUnit=m  TranslationStandardAxis=+Z  TranslationStandardOffset=0  TranslationCartesianOffset=constraint.loc  TranslationROffset=0  TranslationROffsetUnits=m  TranslationZOffset=0  TranslationZOffsetUnits=m  TranslationThetaOffset=0  TranslationThetaOffsetUnits=deg  RotationMethod=None  RotationAngleUnits=deg  RotationStandardAxis=+X  RotationAngle=90  RotationArbitraryAxis=[0 0 1]  FollAlignAxisA=+X  BaseAlignAxisA=+Y  FollAlignAxisB=+Y  BaseAlignAxisB=+Z  RotationMatrix=[1 0 0; 0 1 0; 0 0 1]  BlockFunction=simmechanics.library.frames_transforms.rigid_transform
  Selector : Selector  InputPortWidth=6
  Selector2 : Selector  InputPortWidth=6  Indices=3
  Selector6 : Selector  InputPortWidth=6  Indices=5
  Selector7 : Selector  InputPortWidth=6  Indices=2
  Selector8 : Selector  InputPortWidth=6  Indices=4
  Selector9 : Selector  InputPortWidth=6  Indices=6
  Simulink-PS Converter{1..6} (6 alike) : nesl_utility/Simulink-PS Converter  PhysicalDomain=network_engine_domain  SubClassName=ps_input  LeftPortType=input  RightPortType=output  PseudoPeriodic=off  Frequencies=[]  NoiseDistribution=none  NoiseParameters=[]  Unit=1  AffineConversion=off  InputFiltering=off  SimscapeFilterOrder=1  InputFilterTimeConstant=0.001  UdotUserProvided=1
  output : ToWorkspace  VariableName=constraint1_out  SaveFormat=Structure With Time  SampleTime=-1
      settings: Decimation=round(simu.dtOut/simu.dt,0)
  B : PMIOPort  Port=1  Side=Left
  F : PMIOPort  Port=2  Side=Right
  wires:
  PS-Simulink Converter2/1 -> Mux4/6
  PS-Simulink Converter3/1 -> Mux3/6
  PS-Simulink Converter4/1 -> Mux2/6
  PS-Simulink Converter5/1 -> Mux4/5
  PS-Simulink Converter6/1 -> Mux3/5
  PS-Simulink Converter7/1 -> Mux2/5
  PS-Simulink Converter8/1 -> Mux4/4
  PS-Simulink Converter9/1 -> Mux3/4
  PS-Simulink Converter10/1 -> Mux2/4
  PS-Simulink Converter11/1 -> Mux4/3
  PS-Simulink Converter14/1 -> Mux4/2
  PS-Simulink Converter17/1 -> Mux4/1
  PS-Simulink Converter12/1 -> Mux3/3
  PS-Simulink Converter15/1 -> Mux3/2
  PS-Simulink Converter18/1 -> Mux3/1
  PS-Simulink Converter13/1 -> Mux2/3
  PS-Simulink Converter16/1 -> Mux2/2
  PS-Simulink Converter19/1 -> Mux2/1
  Mux4/1 -> Mux1/3  "acceleration"
  Mux3/1 -> Mooring/3(Velocity), Mux1/2  "velocity"
  Mux2/1 -> Add/1, Mux1/1  "position"
  Mux1/1 -> output/1
  Mux/1 -> Mux1/5  "Constraint Forces"
  PS-Simulink Converter1/1 -> Mux/2
  PS-Simulink Converter/1 -> Mux/1
  Mooring/1(F_Mooring) -> Selector7/1, Selector/1, Selector2/1, Selector8/1, Selector9/1, Selector6/1
  Selector/1 -> Simulink-PS Converter1/1
  Selector2/1 -> Simulink-PS Converter2/1
  Selector6/1 -> Simulink-PS Converter3/1
  [Clock] -> Mooring/2(Clock)
  Selector7/1 -> Simulink-PS Converter4/1
  Selector8/1 -> Simulink-PS Converter5/1
  Selector9/1 -> Simulink-PS Converter6/1
  PS-Simulink Converter21/1 -> Mux5/2
  PS-Simulink Converter20/1 -> Mux5/1
  Mux5/1 -> Mux1/4  "Total Forces"
  Mux6/1 -> Mux1/6  "Mooring Forces"
  PS-Simulink Converter22/1 -> Mux6/6
  PS-Simulink Converter23/1 -> Mux6/5
  PS-Simulink Converter24/1 -> Mux6/4
  PS-Simulink Converter25/1 -> Mux6/3
  PS-Simulink Converter26/1 -> Mux6/2
  PS-Simulink Converter27/1 -> Mux6/1
  Initial Displacement and Angle/1 -> Add/2
  Add/1 -> Mooring/1(Displacement)
  connections:
  Bushing Joint/RConn1 -- Rigid Transform1/RConn1
  Bushing Joint/LConn1 -- Rigid Transform/RConn1
  Rigid Transform1/LConn1 -- F/RConn1
  B/RConn1 -- Rigid Transform/LConn1
  Simulink-PS Converter6/RConn1 -- Bushing Joint/LConn7
  Simulink-PS Converter3/RConn1 -- Bushing Joint/LConn6
  Simulink-PS Converter5/RConn1 -- Bushing Joint/LConn5
  Simulink-PS Converter2/RConn1 -- Bushing Joint/LConn4
  Simulink-PS Converter4/RConn1 -- Bushing Joint/LConn3
  Simulink-PS Converter1/RConn1 -- Bushing Joint/LConn2
  PS-Simulink Converter17/LConn1 -- Bushing Joint/RConn4
  Bushing Joint/RConn3 -- PS-Simulink Converter18/LConn1
  Bushing Joint/RConn2 -- PS-Simulink Converter19/LConn1
  PS-Simulink Converter16/LConn1 -- Bushing Joint/RConn6
  PS-Simulink Converter15/LConn1 -- Bushing Joint/RConn7
  PS-Simulink Converter14/LConn1 -- Bushing Joint/RConn8
  Bushing Joint/RConn10 -- PS-Simulink Converter13/LConn1
  PS-Simulink Converter12/LConn1 -- Bushing Joint/RConn11
  Bushing Joint/RConn12 -- PS-Simulink Converter11/LConn1
  PS-Simulink Converter10/LConn1 -- Bushing Joint/RConn14
  PS-Simulink Converter9/LConn1 -- Bushing Joint/RConn15
  PS-Simulink Converter8/LConn1 -- Bushing Joint/RConn16
  PS-Simulink Converter7/LConn1 -- Bushing Joint/RConn18
  PS-Simulink Converter6/LConn1 -- Bushing Joint/RConn19
  PS-Simulink Converter5/LConn1 -- Bushing Joint/RConn20
  PS-Simulink Converter4/LConn1 -- Bushing Joint/RConn22
  PS-Simulink Converter3/LConn1 -- Bushing Joint/RConn23
  PS-Simulink Converter2/LConn1 -- Bushing Joint/RConn24
  PS-Simulink Converter/LConn1 -- Bushing Joint/RConn26
  Bushing Joint/RConn27 -- PS-Simulink Converter1/LConn1
  PS-Simulink Converter21/LConn1 -- Bushing Joint/RConn29
  PS-Simulink Converter20/LConn1 -- Bushing Joint/RConn28
  PS-Simulink Converter22/LConn1 -- Bushing Joint/RConn25
  Bushing Joint/RConn21 -- PS-Simulink Converter23/LConn1
  Bushing Joint/RConn17 -- PS-Simulink Converter24/LConn1
  Bushing Joint/RConn13 -- PS-Simulink Converter25/LConn1
  PS-Simulink Converter26/LConn1 -- Bushing Joint/RConn9
  Bushing Joint/RConn5 -- PS-Simulink Converter27/LConn1
